simulink model "BLDC_PIL_Sensorless_top"  (R2026a)
settings: Solver=FixedStepDiscrete  StopTime=4  FixedStep=6.25e-5
undefined symbols (not defined in the file or in its folder): BldcPlant_Params
settings Model: DataDictionary=BldcData.sldd  Creator=k  LastModifiedBy=k

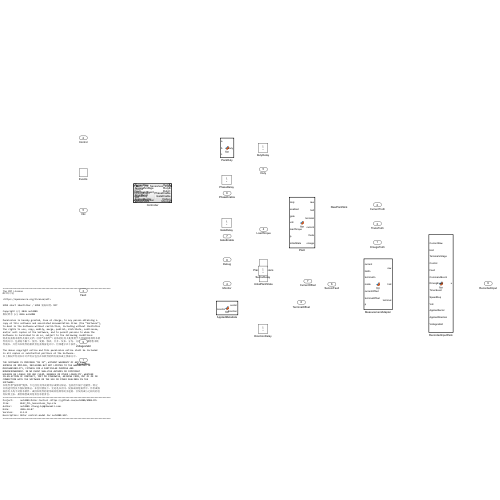
[thumbnail: Simulink's stored preview of the top-level diagram]
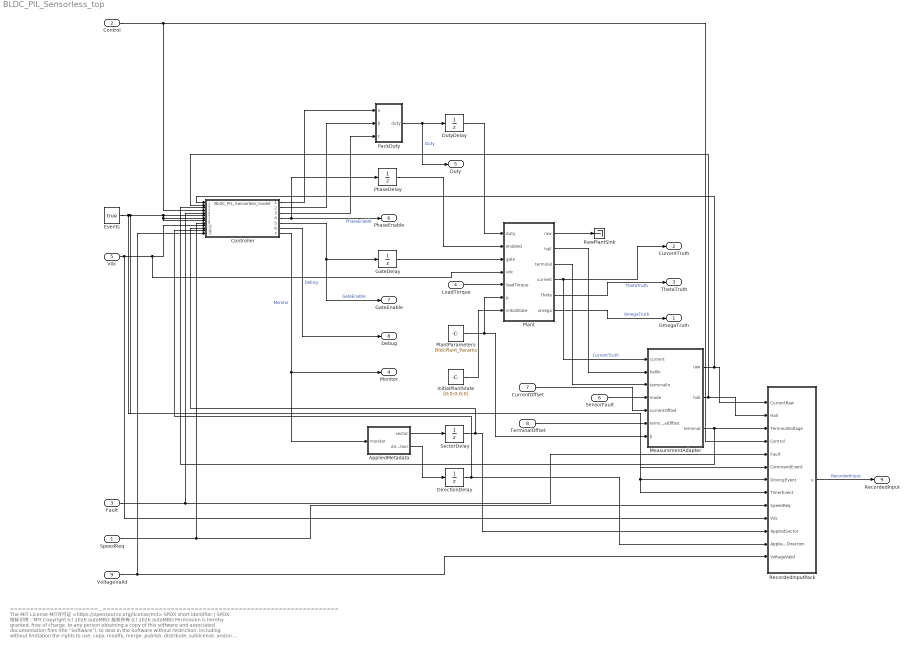
== system BLDC_PIL_Sensorless_top ==
  note: =================================================================================
      | The MIT License
      | MIT许可证
      |
      | <https://opensource.org/license/mit>
      |
      | SPDX short identifier / SPDX 短标识符：MIT
      |
      | Copyright (c) 2026 autoMBD
      | 版权所有 (c) 2026 autoMBD
      |
      | Permission is hereby granted, free of charge, to any person obtaining a
      | copy of this software and associated documentation files (the “Software”),
      | to deal in the Software without restriction, including without limitation
      | the rights to use, copy, modify, merge, publish, distribute, sublicense,
      | and/or sell copies of the Software, and to permit persons to whom the
      | Software is furnished to do so, subject to the following conditions:
      | 特此向获得本软件及相关文档（合称“本软件”）副本的任何人免费授予不受限制地利用本软
      | 件的许可，包括而不限于：使用、复制、修改、合并、发布、分发、分许可和/或销售本软
      | 件副本，并允许本软件的接收者也获得前述许可，但须遵守以下条件：
      |
      | The above copyright notice and this permission notice shall be included
      | in all copies or substantial portions of the Software.
      | 以上版权声明及本许可声明应包含在本软件的所有副本或主要部分中。
      |
      | THE SOFTWARE IS PROVIDED “AS IS”, WITHOUT WARRANTY OF ANY KIND,
      | EXPRESS OR IMPLIED, INCLUDING BUT NOT LIMITED TO THE WARRANTIES OF
      | MERCHANTABILITY, FITNESS FOR A PARTICULAR PURPOSE AND
      | NONINFRINGEMENT. IN NO EVENT SHALLTHE AUTHORS OR COPYRIGHT
      | HOLDERS BE LIABLE FOR ANY CLAIM, DAMAGES OR OTHER LIABILITY, WHETHER
      | IN AN ACTION OF CONTRACT, TORT OR OTHERWISE, ARISING FROM, OUT OF OR IN
      | CONNECTION WITH THE SOFTWARE OR THE USE OR OTHER DEALINGS IN THE
      | SOFTWARE.
      | 本软件系“按原样”提供，不包含任何形式的明示或默示保证，包括但不限于适销性、特定
      | 目的适用性及不侵权的保证。在任何情况下，无论是在合同、侵权或其他案件中，作者或版
      | 权持有人均不对因本软件、或因本软件的使用或其他利用而引起的、引发的或与之相关的任
      | 何权利主张、损害赔偿或其他责任承担责任。
      | =================================================================================
      | Project:     autoMBD Motor Control <https://github.com/autoMBD/AMBD-MC>
      | File:        BLDC_PIL_Sensorless_top.slx
      | Author:      autoMBD <tkung.lqk@foxmail.com>
      | Date:        2026-10-07
      | Version:     0.1.0
      | Description: Motor control model for autoMBD HSP.
      | =================================================================================
  SpeedReq : Inport  OutDataTypeStr=single  PortDimensions=1  SampleTime=6.25e-5
  Control : Inport  Port=2  OutDataTypeStr=uint8  PortDimensions=1  SampleTime=6.25e-5
  Fault : Inport  Port=3  OutDataTypeStr=boolean  PortDimensions=1  SampleTime=6.25e-5
  LoadTorque : Inport  Port=4  OutDataTypeStr=double  PortDimensions=1  SampleTime=6.25e-5
  Vdc : Inport  Port=5  OutDataTypeStr=single  PortDimensions=1  SampleTime=6.25e-5
  SensorFault : Inport  Port=6  OutDataTypeStr=uint8  PortDimensions=1  SampleTime=6.25e-5
  CurrentOffset : Inport  Port=7  OutDataTypeStr=single  PortDimensions=3  SampleTime=6.25e-5
  TerminalOffset : Inport  Port=8  OutDataTypeStr=single  PortDimensions=3  SampleTime=6.25e-5
  VoltageValid : Inport  Port=9  OutDataTypeStr=boolean  PortDimensions=1  SampleTime=6.25e-5
  AppliedMetadata : MATLAB Function  TreatAsAtomicUnit=on
  Controller : ModelReference  ModelNameDialog=BLDC_PIL_Sensorless_model  SimulationMode=Normal  CodeInterface=Top model  ModelReferenceVersion=1.2
  DirectionDelay : UnitDelay  InitialCondition=int8(1)  SampleTime=6.25e-5
  DutyDelay : UnitDelay  InitialCondition=uint16([0;0;0])  SampleTime=6.25e-5
  Events : Constant  Value=true  OutDataTypeStr=boolean
  GateDelay : UnitDelay  InitialCondition=false  SampleTime=6.25e-5
  InitialPlantState : Constant  Value=[0;0;0;0;0]  OutDataTypeStr=double
  MeasurementAdapter : MATLAB Function  TreatAsAtomicUnit=on
  PackDuty : MATLAB Function  TreatAsAtomicUnit=on
  PhaseDelay : UnitDelay  InitialCondition=false(3,1)  SampleTime=6.25e-5
  Plant : MATLAB Function  TreatAsAtomicUnit=on
  PlantParameters : Constant  Value=BldcPlant_Params  OutDataTypeStr=Bus: tBldcParams
  RawPlantSink : Terminator
  RecordedInputPack : MATLAB Function  TreatAsAtomicUnit=on
  SectorDelay : UnitDelay  InitialCondition=uint8(0)  SampleTime=6.25e-5
  OmegaTruth : Outport  OutDataTypeStr=single  PortDimensions=1
  CurrentTruth : Outport  Port=2  OutDataTypeStr=single  PortDimensions=3
  ThetaTruth : Outport  Port=3  OutDataTypeStr=single  PortDimensions=1
  Monitor : Outport  Port=4  OutDataTypeStr=Bus: tBldcMonitor  PortDimensions=1
  Duty : Outport  Port=5  OutDataTypeStr=uint16  PortDimensions=3
  PhaseEnable : Outport  Port=6  OutDataTypeStr=boolean  PortDimensions=3
  GateEnable : Outport  Port=7  OutDataTypeStr=boolean  PortDimensions=1
  Debug : Outport  Port=8  OutDataTypeStr=Bus: tBldcDebug  PortDimensions=1
  RecordedInput : Outport  Port=9  OutDataTypeStr=Bus: tBldcInput  PortDimensions=1
  wires:
  VoltageValid/1 -> Controller/13, RecordedInputPack/13(VoltageValid)
  DirectionDelay/1 -> Controller/12, RecordedInputPack/12(AppliedDirection)
  SectorDelay/1 -> RecordedInputPack/11(AppliedSector), Controller/11
  SpeedReq/1 -> Controller/9, RecordedInputPack/9(SpeedReq)
  Events/1 -> RecordedInputPack/8(TimerEvent), RecordedInputPack/7(DrivingEvent), Controller/8, Controller/7, Controller/6, RecordedInputPack/6(CommandEvent)
  Fault/1 -> Controller/5, RecordedInputPack/5(Fault)
  Control/1 -> Controller/4, RecordedInputPack/4(Control)
  MeasurementAdapter/3(terminal) -> RecordedInputPack/3(TerminalVoltage), Controller/3
  MeasurementAdapter/2(hall) -> Controller/2, RecordedInputPack/2(Hall)
  MeasurementAdapter/1(raw) -> Controller/1, RecordedInputPack/1(CurrentRaw)
  InitialPlantState/1 -> Plant/7(initialState)
  Controller/3 -> PackDuty/3(c)
  Controller/2 -> PackDuty/2(b)
  Controller/1 -> PackDuty/1(a)
  RecordedInputPack/1(u) -> RecordedInput/1  "RecordedInput"
  AppliedMetadata/2(direction) -> DirectionDelay/1
  AppliedMetadata/1(sector) -> SectorDelay/1
  Controller/7 -> AppliedMetadata/1(monitor), Monitor/1  "Monitor"
  Controller/6 -> Debug/1  "Debug"
  Controller/5 -> GateDelay/1, GateEnable/1  "GateEnable"
  Controller/4 -> PhaseDelay/1, PhaseEnable/1  "PhaseEnable"
  PackDuty/1(duty) -> DutyDelay/1, Duty/1  "Duty"
  Plant/5(theta) -> ThetaTruth/1  "ThetaTruth"
  Plant/6(omega) -> OmegaTruth/1  "OmegaTruth"
  TerminalOffset/1 -> MeasurementAdapter/6(terminalOffset)
  CurrentOffset/1 -> MeasurementAdapter/5(currentOffset)
  SensorFault/1 -> MeasurementAdapter/4(mode)
  Plant/3(terminal) -> MeasurementAdapter/3(terminalIn)
  Plant/2(hall) -> MeasurementAdapter/2(hallIn)
  Plant/4(current) -> CurrentTruth/1, MeasurementAdapter/1(current)  "CurrentTruth"
  Plant/1(raw) -> RawPlantSink/1
  PlantParameters/1 -> Plant/6(p), MeasurementAdapter/7(p)
  LoadTorque/1 -> Plant/5(loadTorque)
  Vdc/1 -> Controller/10, Plant/4(vdc), RecordedInputPack/10(Vdc)
  GateDelay/1 -> Plant/3(gate)
  PhaseDelay/1 -> Plant/2(enabled)
  DutyDelay/1 -> Plant/1(duty)

== matlab function BLDC_PIL_Sensorless_top/MeasurementAdapter ==
  data: current input; raw output; hallIn input; terminalIn input; mode input; currentOffset input; terminalOffset input; p input; hall output; terminal output
function [raw,hall,terminal]=fcn(current,hallIn,terminalIn,mode,currentOffset,terminalOffset,p)
%#codegen
persistent state
if isempty(state),state=struct('Hall',uint8(5),'Terminal',repmat(p.NominalVdc/single(2),3,1));end
[raw,hall,terminal,state]=bldc_measurement_adapter(current,hallIn,terminalIn,mode,currentOffset,terminalOffset,p,state);
end

== matlab function BLDC_PIL_Sensorless_top/Plant ==
  data: duty input; raw output; enabled input; gate input; vdc input; loadTorque input; p input; initialState input; hall output; terminal output; current output; theta output; omega output
function [raw,hall,terminal,current,theta,omega]=fcn(duty,enabled,gate,vdc,loadTorque,p,initialState)
%#codegen
persistent x
if isempty(x)
x=initialState;
else
x=bldc.plant_step(x,duty,enabled,gate,vdc,loadTorque,p,6.25e-5);
end
[raw,hall,terminal,current,theta,omega]=bldc.plant_measure(x,duty,enabled,gate,vdc,p);
end

== matlab function BLDC_PIL_Sensorless_top/PackDuty ==
  data: a input; duty output; b input; c input
function duty=fcn(a,b,c)
%#codegen
duty=[a;b;c];
end

== matlab function BLDC_PIL_Sensorless_top/AppliedMetadata ==
  data: monitor input; sector output; direction output
function [sector,direction]=fcn(monitor)
%#codegen
sector=uint8(0);if monitor.GateEnable,sector=monitor.Sector;end
direction=monitor.OutputDirection;
end

== matlab function BLDC_PIL_Sensorless_top/RecordedInputPack ==
  data: CurrentRaw input; u output Bus: tBldcInput; Hall input; TerminalVoltage input; Control input; Fault input; CommandEvent input; DrivingEvent input; TimerEvent input; SpeedReq input; Vdc input; AppliedSector input; AppliedDirection input; VoltageValid input
function u=fcn(CurrentRaw,Hall,TerminalVoltage,Control,Fault,CommandEvent,DrivingEvent,TimerEvent,SpeedReq,Vdc,AppliedSector,AppliedDirection,VoltageValid)
%#codegen
u.CurrentRaw=CurrentRaw;
u.Hall=Hall;
u.TerminalVoltage=TerminalVoltage;
u.Control=Control;
u.Fault=Fault;
u.CommandEvent=CommandEvent;
u.DrivingEvent=DrivingEvent;
u.TimerEvent=TimerEvent;
u.SpeedReq=SpeedReq;
u.Vdc=Vdc;
u.AppliedSector=AppliedSector;
u.AppliedDirection=AppliedDirection;
u.VoltageValid=VoltageValid;
end
